simulink model "Digital-Memory-Architecture"  (R2024b)
settings: Solver=VariableStepAuto  StartTime=0.0  StopTime=10.0  RelTol=1e-3
libraries: simulink_extras x129
(part 5 of 5)

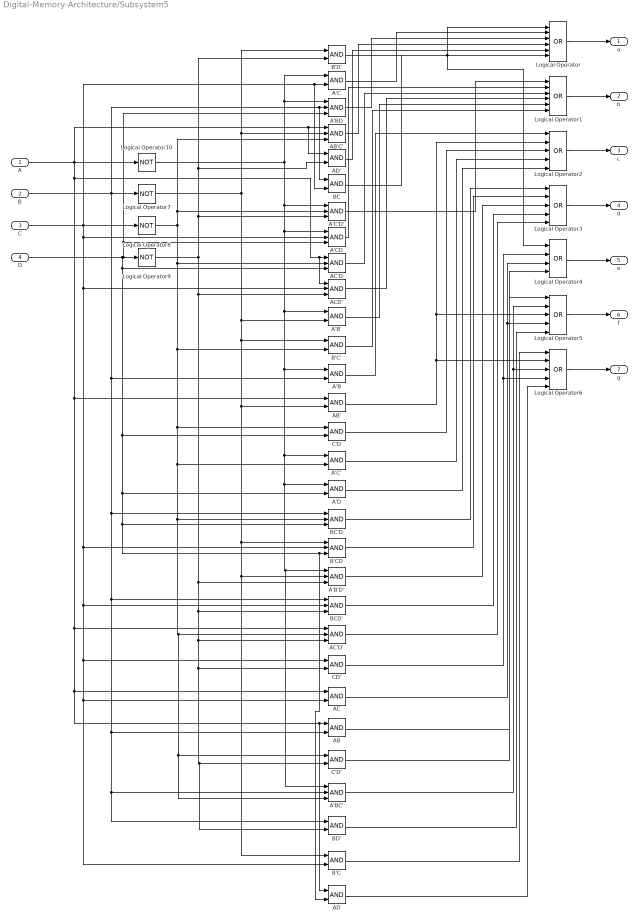
== system Digital-Memory-Architecture/Subsystem5 ==
  A : Inport
  B : Inport  Port=2
  C : Inport  Port=3
  D : Inport  Port=4
  A'B : Logic  AllPortsSameDT=off  OutDataTypeStr=boolean
  A'B' : Logic  AllPortsSameDT=off  OutDataTypeStr=boolean
  A'B'D' : Logic  Inputs=3  AllPortsSameDT=off  OutDataTypeStr=boolean
  A'BC' : Logic  Inputs=3  AllPortsSameDT=off  OutDataTypeStr=boolean
  A'BD : Logic  Inputs=3  AllPortsSameDT=off  OutDataTypeStr=boolean
  A'C : Logic  AllPortsSameDT=off  OutDataTypeStr=boolean
  A'C' : Logic  AllPortsSameDT=off  OutDataTypeStr=boolean
  A'C'D' : Logic  Inputs=3  AllPortsSameDT=off  OutDataTypeStr=boolean
  A'CD : Logic  Inputs=3  AllPortsSameDT=off  OutDataTypeStr=boolean
  A'D : Logic  AllPortsSameDT=off  OutDataTypeStr=boolean
  AB : Logic  AllPortsSameDT=off  OutDataTypeStr=boolean
  AB' : Logic  AllPortsSameDT=off  OutDataTypeStr=boolean
  AB'C' : Logic  Inputs=3  AllPortsSameDT=off  OutDataTypeStr=boolean
  AC : Logic  AllPortsSameDT=off  OutDataTypeStr=boolean
  AC'D : Logic  Inputs=3  AllPortsSameDT=off  OutDataTypeStr=boolean
  AC'D' : Logic  Inputs=3  AllPortsSameDT=off  OutDataTypeStr=boolean
  ACD' : Logic  Inputs=3  AllPortsSameDT=off  OutDataTypeStr=boolean
  AD : Logic  AllPortsSameDT=off  OutDataTypeStr=boolean
  AD' : Logic  AllPortsSameDT=off  OutDataTypeStr=boolean
  B'C : Logic  AllPortsSameDT=off  OutDataTypeStr=boolean
  B'C' : Logic  AllPortsSameDT=off  OutDataTypeStr=boolean
  B'CD : Logic  Inputs=3  AllPortsSameDT=off  OutDataTypeStr=boolean
  B'D' : Logic  AllPortsSameDT=off  OutDataTypeStr=boolean
  BC : Logic  AllPortsSameDT=off  OutDataTypeStr=boolean
  BC'D : Logic  Inputs=3  AllPortsSameDT=off  OutDataTypeStr=boolean
  BCD' : Logic  Inputs=3  AllPortsSameDT=off  OutDataTypeStr=boolean
  BD' : Logic  AllPortsSameDT=off  OutDataTypeStr=boolean
  C'D : Logic  AllPortsSameDT=off  OutDataTypeStr=boolean
  C'D' : Logic  AllPortsSameDT=off  OutDataTypeStr=boolean
  CD' : Logic  AllPortsSameDT=off  OutDataTypeStr=boolean
  Logical Operator : Logic  Operator=OR  Inputs=6  AllPortsSameDT=off  OutDataTypeStr=boolean
  Logical Operator1 : Logic  Operator=OR  Inputs=6  AllPortsSameDT=off  OutDataTypeStr=boolean
  Logical Operator{7..10} (4 alike) : Logic  Operator=NOT  AllPortsSameDT=off  OutDataTypeStr=boolean
  Logical Operator{2..3,5..6} (4 alike) : Logic  Operator=OR  Inputs=5  AllPortsSameDT=off  OutDataTypeStr=boolean
  Logical Operator4 : Logic  Operator=OR  Inputs=4  AllPortsSameDT=off  OutDataTypeStr=boolean
  a : Outport
  b : Outport  Port=2
  c : Outport  Port=3
  d : Outport  Port=4
  e : Outport  Port=5
  f : Outport  Port=6
  g : Outport  Port=7
  wires:
  Logical Operator6/1 -> g/1
  Logical Operator5/1 -> f/1
  Logical Operator4/1 -> e/1
  Logical Operator3/1 -> d/1
  Logical Operator2/1 -> c/1
  Logical Operator1/1 -> b/1
  Logical Operator/1 -> a/1
  B/1 -> BD'/1, A'BC'/2, AB/2, BCD'/1, BC'D/1, A'B/2, Logical Operator7/1, BC/1, A'BD/2
  D/1 -> AD/2, B'CD/3, BC'D/3, A'D/2, C'D/2, AC'D/3, A'BD/3, A'CD/3, Logical Operator9/1
  Logical Operator7/1 -> B'C/1, A'B'D'/2, B'CD/1, AB'/2, B'C'/1, A'B'/2, AB'C'/2, B'D'/1
  Logical Operator9/1 -> BD'/2, C'D'/2, CD'/2, AC'D'/3, BCD'/3, A'B'D'/3, ACD'/3, AD'/2, B'D'/2, A'C'D'/3
  B'D'/1 -> Logical Operator4/1, Logical Operator/1
  A/1 -> AD/1, AB/1, AC/1, AC'D'/1, AB'/1, ACD'/1, AC'D/1, AD'/1, AB'C'/1, Logical Operator10/1
  Logical Operator10/1 -> A'BC'/1, A'B'D'/1, A'D/1, A'C'/1, A'B/1, A'B'/1, A'CD/1, A'C'D'/1, A'BD/1, A'C/1
  C/1 -> B'C/2, AC/2, CD'/1, BCD'/2, B'CD/2, ACD'/2, A'CD/2, Logical Operator8/1, BC/2, A'C/2
  A'C/1 -> Logical Operator/2
  A'BD/1 -> Logical Operator/3
  Logical Operator8/1 -> A'BC'/3, C'D'/1, AC'D'/2, BC'D/2, A'C'/2, C'D/1, B'C'/2, AC'D/2, A'C'D'/2, AB'C'/3
  AB'C'/1 -> Logical Operator/4
  AD'/1 -> Logical Operator/5
  BC/1 -> Logical Operator/6
  A'C'D'/1 -> Logical Operator1/1
  A'CD/1 -> Logical Operator1/2
  AC'D/1 -> Logical Operator1/3
  ACD'/1 -> Logical Operator1/4
  A'B'/1 -> Logical Operator1/5
  B'C'/1 -> Logical Operator1/6
  A'B/1 -> Logical Operator2/1
  AB'/1 -> Logical Operator6/2, Logical Operator5/3, Logical Operator2/2
  C'D/1 -> Logical Operator2/3
  A'C'/1 -> Logical Operator2/4
  A'D/1 -> Logical Operator2/5
  BC'D/1 -> Logical Operator3/1
  B'CD/1 -> Logical Operator3/2
  A'B'D'/1 -> Logical Operator3/3
  BCD'/1 -> Logical Operator3/4
  AC'D'/1 -> Logical Operator3/5
  CD'/1 -> Logical Operator6/4, Logical Operator4/2
  AC/1 -> Logical Operator5/4, Logical Operator4/3
  AB/1 -> Logical Operator4/4
  C'D'/1 -> Logical Operator5/1
  A'BC'/1 -> Logical Operator6/3, Logical Operator5/2
  BD'/1 -> Logical Operator5/5
  B'C/1 -> Logical Operator6/1
  AD/1 -> Logical Operator6/5
